simulink model "MODELODETURBINADERIOV5"  (R2017a)
settings: Solver=ode45  StartTime=0.0  StopTime=0.05  FixedStep=50e-3  MaxStep=0.01  RelTol=1e-3
values from neighbouring files (symbols this model uses):
  A = pi()*((D/2)^2)    [MODELOHIDRO.m]    (also in MODELOHIDROV10.m; MODELOHIDROV2.m; MODELOHIDROV3.m; MODELOHIDROV4.m)
  B = 0    [MODELOHIDRO.m]    (also in MODELOHIDROV10.m; MODELOHIDROV2.m; MODELOHIDROV3.m; MODELOHIDROV4.m)
  beta = 0    [MODELOHIDRO.m]    (also in MODELOHIDROV10.m; MODELOHIDROV2.m; MODELOHIDROV3.m; MODELOHIDROV4.m)
  Bi = 0.2287    [MODELOHIDRO.m]    (also in MODELOHIDROV10.m = 0.1; MODELOHIDROV2.m; MODELOHIDROV3.m; MODELOHIDROV4.m = 0.005)
  den = 1000    [MODELOHIDRO.m]    (also in MODELOHIDROV10.m; MODELOHIDROV2.m; MODELOHIDROV3.m; MODELOHIDROV4.m)
  J = 16.1919e-4    (= 0.00161919)    [MODELOHIDROV10.m]    (also in MODELOHIDROV2.m = 100; MODELOHIDROV3.m = 10; MODELOHIDROV4.m; MODELOHIDROV7.m)
  Ji = 1    [MODELOHIDRO.m]    (also in MODELOHIDROV10.m = 1.72; MODELOHIDROV2.m; MODELOHIDROV3.m; MODELOHIDROV4.m = 0.0465)
  Kb = 1.8    [MODELOHIDRO.m]    (also in MODELOHIDROV10.m = 6.2; MODELOHIDROV2.m; MODELOHIDROV3.m; MODELOHIDROV4.m = 0.027)
  Kp = 0.4    [MODELOHIDRO.m]    (also in MODELOHIDROV10.m = 5.6627; MODELOHIDROV2.m; MODELOHIDROV3.m; MODELOHIDROV4.m = 0.027)
  L_d = 38e-3    (= 0.038)    [MODELOHIDROV2.m]    (also in MODELOHIDROV3.m; MODELOHIDROV4.m; MODELOHIDROV7.m)
  L_q = 9.03e-3    (= 0.00903)    [MODELOHIDROV2.m]    (also in MODELOHIDROV3.m; MODELOHIDROV4.m; MODELOHIDROV7.m)
  Lambda = 0.48    [MODELOHIDROV2.m]    (also in MODELOHIDROV3.m; MODELOHIDROV4.m; MODELOHIDROV7.m)
  P = 1    [MODELOHIDROV2.m]    (also in MODELOHIDROV3.m; MODELOHIDROV4.m; MODELOHIDROV7.m)
  r = D/2    (= 0.5)    [MODELOHIDRO.m]    (also in MODELOHIDROV10.m; MODELOHIDROV2.m; MODELOHIDROV3.m; MODELOHIDROV4.m)
  Ri = 0.6    [MODELOHIDRO.m]    (also in MODELOHIDROV10.m = 0.973; MODELOHIDROV2.m; MODELOHIDROV3.m; MODELOHIDROV4.m = 1)
  Rs = 1.649    [MODELOHIDROV2.m]    (also in MODELOHIDROV3.m; MODELOHIDROV4.m; MODELOHIDROV7.m)
  T_d = 0    [MODELOHIDRO.m]    (also in MODELOHIDROV10.m; MODELOHIDROV2.m; MODELOHIDROV3.m; MODELOHIDROV4.m)
undefined symbols (not defined in the file or in its folder): sigbuilder_block
libraries: powerlib x19, simulink x2
settings Model: Creator=zni.uao  LastModifiedBy=zni.uao
settings SolverCC: ZeroCrossAlgorithm=Adaptive
settings OptimizationCC: LifeSpan=inf
settings HardwareCC: ProdBitPerPointer=32  ProdBitPerSizeT=32  ProdBitPerPtrDiffT=32  ProdLargestAtomicFloat=None  ProdWordSize=32  ProdHWDeviceType=Custom Processor->Custom

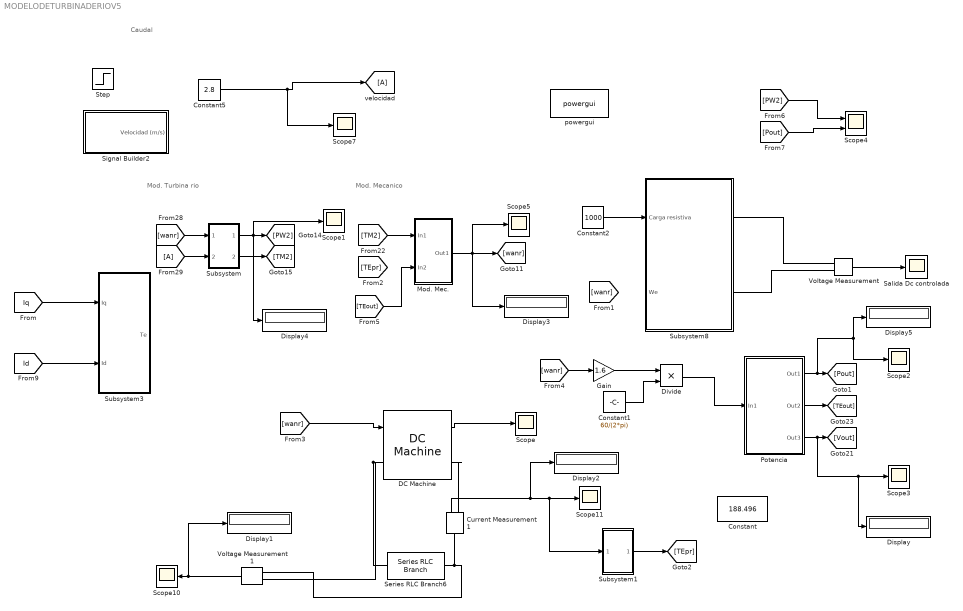
== system MODELODETURBINADERIOV5 ==
  note: Mod. Turbina rio
  note: Mod. Mecanico
  note: Caudal
  Constant : Constant  Value=188.496
  Constant1 : Constant  Value=60/(2*pi)
  Constant2 : Constant  Value=1000
  Constant5 : Constant  Value=2.8
  Current Measurement1 : powerlib/Measurements/Current Measurement  PhasorSimulation=off  OutputType=Complex  PSBequivalent=0
  DC Machine : powerlib/Machines/DC Machine  PresetModel=No  MechanicalLoad=Speed w  FieldType=Permanent magnet  ShowDetailedParameters=on  MeasurementBus=off  RLa=[0.78 0.016]  RLf=[150 112.5]  Laf=1.234  MachineConstant=Torque constant (N.m/A)  Ke=1.8  Kt=1.8  J=0.05  Bm=0.01  Tf=0  w0=1  Ifinit=1  TsPowergui=0  TsBlock=-1
  Display{,1..5} (6 alike) : Display
  Divide : Product  Inputs=**
  Gain : Gain  Gain=1.6
  Mod. Mec. : Subsystem
  Potencia : Subsystem
  Salida Dc controlada : Scope
  Scope{,1..3,5,7,10..11} (8 alike) : Scope
  Scope4 : Scope  NumInputPorts=2
  Series RLC Branch6 : powerlib/Elements/Series RLC Branch  LConnTagsString=__new0  RConnTagsString=__new0  BranchType=R  Resistance=1000  Inductance=1e-3  SetiL0=off  InitialCurrent=0  Capacitance=1e-6  Setx0=off  InitialVoltage=0  Measurements=None
  Signal Builder2 : Subsystem  Tag=STV Subsys  LoadFcn=sigbuilder_block('load');  StartFcn=sigbuilder_block('start');  StopFcn=sigbuilder_block('stop');  ClipboardFcn=sigbuilder_block('clipboard');  mask(Sigbuilder block){tuvar=[0:10]}
      mask help: Simulink:masks:SigbuilderBlock_MD
      mask init:
      | if ~strcmp(get_param(bdroot(gcbh),'SimulationStatus'),'stopped') tuvar = sigbuilder_block('maskInit'); end
      settings: CopyFcn=sigbuilder_block('copy');  DeleteFcn=sigbuilder_block('delete');  ModelCloseFcn=sigbuilder_block('modelClose');  PreSaveFcn=sigbuilder_block('preSave');  PauseFcn=sigbuilder_block('pause');  ContinueFcn=sigbuilder_block('continue');  NameChangeFcn=sigbuilder_block('namechange');  OpenFcn=sigbuilder_block('open',[197.25 66 550.5 359.25 ]);  CloseFcn=sigbuilder_block('close');
      mask Display: plot(0, 0, 100, 100,[2, 2, 32, 32, 2], [68, 8, 8, 68, 68],[32, 2], [38, 38], [32, 19, 2],[53, 60, 44], [32, 17, 17, 2],[16, 16, 31, 31]);txt = getActiveGroup(gcbh);text(2, 100, txt,'verticalAlignment', 'top');
  Step : Step  Time=10  Before=2.5  After=2.888  SampleTime=0
  Subsystem : Subsystem
  Subsystem1 : Subsystem
  Subsystem3 : Subsystem
  Subsystem8 : Subsystem
  Voltage Measurement : powerlib/Measurements/Voltage Measurement  PhasorSimulation=off  OutputType=Complex  PSBequivalent=0
  Voltage Measurement1 : powerlib/Measurements/Voltage Measurement  PhasorSimulation=off  OutputType=Complex  PSBequivalent=0
  powergui : powerlib/powergui  Priority=1  SimulationMode=Continuous  SampleTime=50e-3  frequency=60  Iterations=50  frequencyindice=0  Pbase=100e6  ErrMax=1e-4  UnitsV=kV  UnitsW=MW  buscounter=0  FunctionMessages=off  echomessages=off  EnableUseOfTLC=off  CurrentSourceSwitches=off  DisableSnubberDevices=off  DisableRonSwitches=off  DisableVfSwitches=off  DisplayEquations=off  SolverType=Tustin/Backward Euler (TBE)  Interpol=off  ExternalGateDelay=off  methode=off  Ts=100  x0status=blocks  SPID=off  SwTol=0  HookPort=off  RestoreLinks=warning  ResistiveCurrentMeasurement=off  Frange=[0:2:500]  Ylog=off  Xlog=on  ShowGrid=off  save=off  variable=ZData  structure=0  ZoomFFT=off  StartTime=0.0  cycles=1  DisplayStyle=1  fundamental=60  FreqAxis=off  MaxFrequency=1000  frequencyindicesteady=0 Hz  RmsSteady=1  display=off
  wires:
  [wanr] -> Subsystem/1(In1)
  [A] -> Subsystem/2(In2)
  Subsystem/1(Out1) -> Display4/1, Scope1/1, [PW2]
  Subsystem/2(Out2) -> [TM2]
  Mod. Mec./1(Out1) -> Display3/1, Scope5/1, [wanr]
  [TM2] -> Mod. Mec./1(In1)
  [Iq] -> Subsystem3/1(Iq)
  [Id] -> Subsystem3/2(Id)
  Constant2/1 -> Subsystem8/1(Carga resistiva)
  Voltage Measurement/1 -> Salida Dc controlada/1
  [wanr] -> DC Machine/1
  Voltage Measurement1/1 -> Display1/1, Scope10/1
  DC Machine/1 -> Scope/1
  Current Measurement1/1 -> Display2/1, Subsystem1/1(In1), Scope11/1
  Subsystem1/1(Out1) -> [TEpr]
  Potencia/1(Out1) -> Display5/1, Scope2/1, [Pout]
  Potencia/3(Out3) -> Display/1, Scope3/1, [Vout]
  Potencia/2(Out2) -> [TEout]
  [PW2] -> Scope4/1
  [Pout] -> Scope4/2
  [TEout] -> Mod. Mec./2(In2)
  Constant5/1 -> Scope7/1, [A]
  Gain/1 -> Divide/1
  Constant1/1 -> Divide/2
  Divide/1 -> Potencia/1(In1)
  [wanr] -> Gain/1
  connections:
  Subsystem8/RConn2 -- Voltage Measurement/LConn2
  Subsystem8/RConn1 -- Voltage Measurement/LConn1
  Current Measurement1/LConn1 -- Series RLC Branch6/RConn1 -- Voltage Measurement1/LConn2
  DC Machine/LConn1 -- Series RLC Branch6/LConn1 -- Voltage Measurement1/LConn1
  DC Machine/RConn1 -- Current Measurement1/RConn1

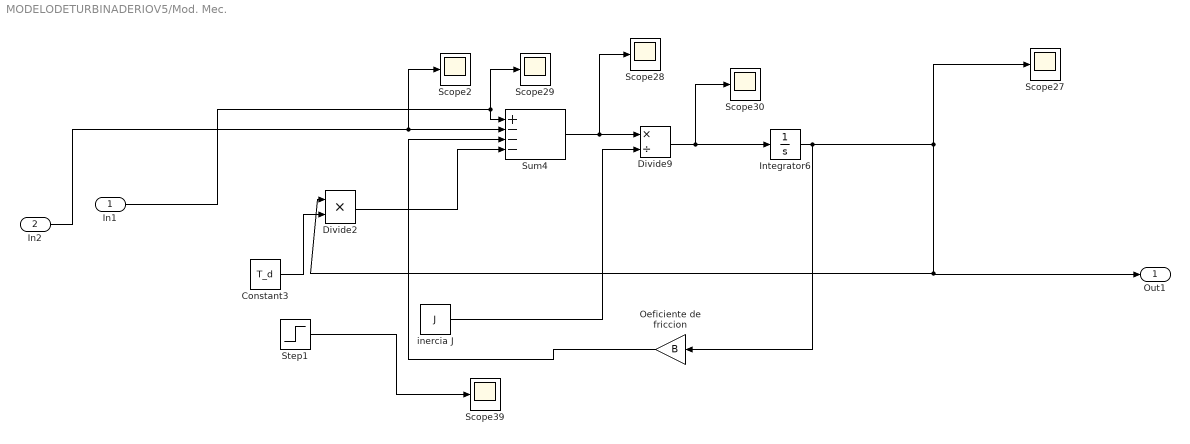
== system MODELODETURBINADERIOV5/Mod. Mec. ==
  In1 : Inport
  In2 : Inport  Port=2
  Constant3 : Constant  Value=T_d
  Divide2 : Product  Inputs=**
  Divide9 : Product  Inputs=*/
  Integrator6 : Integrator  InitialCondition=10
  Oeficiente de friccion : Gain  Gain=B
  Scope{2,27..30,39} (6 alike) : Scope
  Step1 : Step  Time=3  Before=4  After=0  SampleTime=0
  Sum4 : Sum  Inputs=|+---
  inercia J : Constant  Value=J
  Out1 : Outport
  wires:
  inercia J/1 -> Divide9/2
  Constant3/1 -> Divide2/2
  Divide2/1 -> Sum4/4
  Oeficiente de friccion/1 -> Sum4/3
  Step1/1 -> Scope39/1
  Sum4/1 -> Scope28/1, Divide9/1
  In1/1 -> Scope29/1, Sum4/1
  In2/1 -> Scope2/1, Sum4/2
  Divide9/1 -> Scope30/1, Integrator6/1
  Integrator6/1 -> Out1/1, Divide2/1, Scope27/1, Oeficiente de friccion/1

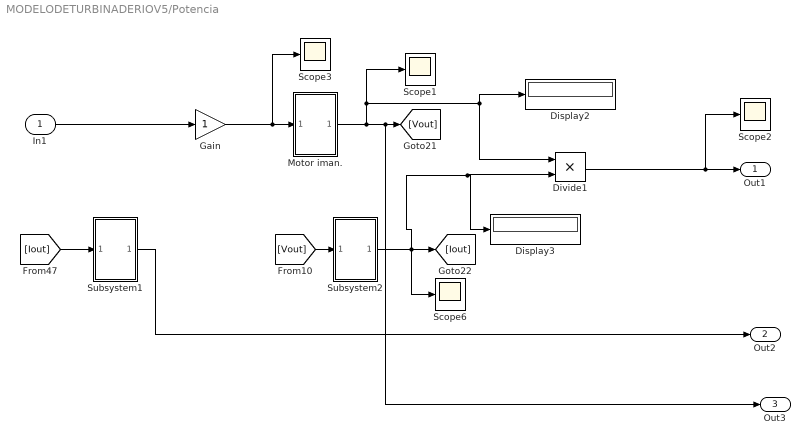
== system MODELODETURBINADERIOV5/Potencia ==
  In1 : Inport
  Display2 : Display
  Display3 : Display
  Divide1 : Product  Inputs=**
  Gain : Gain
  Motor iman. : Subsystem
  Scope{1..3,6} (4 alike) : Scope
  Subsystem1 : Subsystem
  Subsystem2 : Subsystem
  Out1 : Outport
  Out2 : Outport  Port=2
  Out3 : Outport  Port=3
  wires:
  Motor iman./1(Out1) -> Out3/1, [Vout], Scope1/1, Divide1/1, Display2/1
  Subsystem1/1(Out1) -> Out2/1
  [Iout] -> Subsystem1/1(In1)
  Subsystem2/1(Out1) -> Divide1/2, Display3/1, Scope6/1, [Iout]
  Divide1/1 -> Scope2/1, Out1/1
  Gain/1 -> Scope3/1, Motor iman./1(In1)
  In1/1 -> Gain/1
  [Vout] -> Subsystem2/1(In1)

== system MODELODETURBINADERIOV5/Signal Builder2 ==
  Demux : Demux  Tag=STV Demux  Outputs=1
  FromWs : FromWorkspace  Tag=STV FromWs  VariableName=tuvar  SampleTime=0
      SigBuilderData=|
      | common.afterFinalStr = 'Extrapolate'
      | common.sampleTime = 0
      | dataSet.timeRange = [0 0.1]
      | dataSet.name = 'Group 1'
      | sbobj.Groups.Name = 'Group 1'
      | sbobj.Groups.Signals.Name = 'Velocidad (m/s)'
      | sbobj.Groups.Signals.XData = [0 0.01 0.01 0.02 0.02 0.0298 0.0298 0.0398 0.0498 0.06 0.1]
      | sbobj.Groups.Signals.YData = [2 2 2.5 2.5 2.595 2.595 2.8 2.8 2.8 2.8 2.8]
      | sbobj.Groups.TimeRange = [0 0.1]
  Velocidad (m/s) : Outport  Tag=STV Outport
  wires:
  FromWs/1 -> Demux/1
  Demux/1 -> Velocidad (m/s)/1

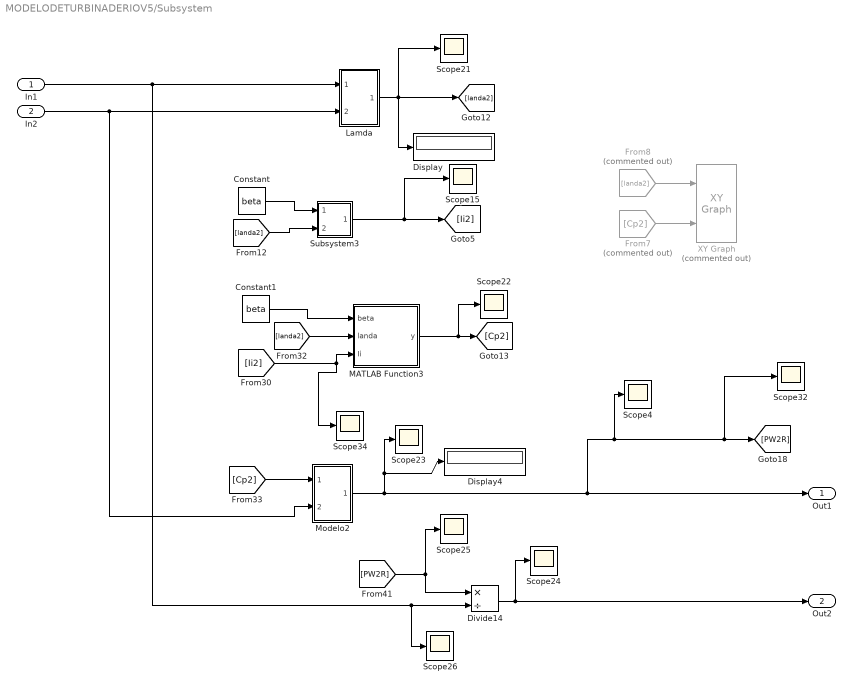
== system MODELODETURBINADERIOV5/Subsystem ==
  In1 : Inport
  In2 : Inport  Port=2
  Constant : Constant  Value=beta
  Constant1 : Constant  Value=beta
  Display : Display
  Display4 : Display
  Divide14 : Product  Inputs=*/
  From7 : From  Commented=on  GotoTag=Cp2
  From8 : From  Commented=on  GotoTag=landa2
  Lamda : Subsystem
  MATLAB Function3 : MATLAB Function  TreatAsAtomicUnit=on
  Modelo2 : Subsystem
  Scope{4,15,21..26,32,34} (10 alike) : Scope
  Subsystem3 : Subsystem
  XY Graph : simulink/Sinks/XY Graph  Commented=on  xmin=1  xmax=20  ymin=0  ymax=0.56  st=0.1
  Out1 : Outport
  Out2 : Outport  Port=2
  wires:
  Constant1/1 -> MATLAB Function3/1(beta)
  Divide14/1 -> Out2/1, Scope24/1
  [Ii2] -> Scope34/1, MATLAB Function3/3(Ii)
  [Cp2] -> Modelo2/1(In1)
  [PW2R] -> Scope25/1, Divide14/1
  In1/1 -> Scope26/1, Divide14/2, Lamda/1(In1)
  [landa2] -> MATLAB Function3/2(landa)
  In2/1 -> Modelo2/2(In2), Lamda/2(In2)
  Lamda/1(Out1) -> Display/1, [landa2], Scope21/1
  MATLAB Function3/1(y) -> Scope22/1, [Cp2]
  From8/1 -> XY Graph/1
  Constant/1 -> Subsystem3/1(In1)
  [landa2] -> Subsystem3/2(In2)
  Modelo2/1(Out1) -> Scope32/1, [PW2R], Scope4/1, Out1/1, Display4/1, Scope23/1
  Subsystem3/1(Out1) -> Scope15/1, [Ii2]
  From7/1 -> XY Graph/2

== system MODELODETURBINADERIOV5/Subsystem1 ==
  In1 : Inport
  Constant2 : Constant  Value=Kp
  Divide2 : Product  Inputs=**
  Out1 : Outport
  wires:
  In1/1 -> Divide2/1
  Constant2/1 -> Divide2/2
  Divide2/1 -> Out1/1

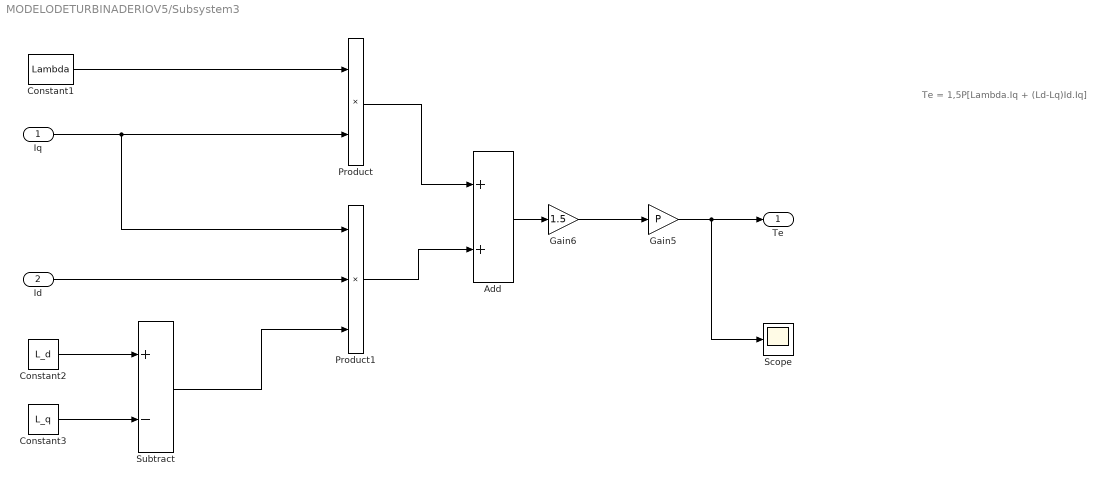
== system MODELODETURBINADERIOV5/Subsystem3 ==
  note: Te = 1,5P[Lambda.Iq + (Ld-Lq)Id.Iq]
  Iq : Inport
  Id : Inport  Port=2
  Add : Sum
  Constant1 : Constant  Value=Lambda
  Constant2 : Constant  Value=L_d
  Constant3 : Constant  Value=L_q
  Gain5 : Gain  Gain=P
  Gain6 : Gain  Gain=1.5
  Product : Product
  Product1 : Product  Inputs=3
  Scope : Scope
  Subtract : Sum  Inputs=+-
  Te : Outport
  wires:
  Product1/1 -> Add/2
  Iq/1 -> Product1/1, Product/2
  Constant1/1 -> Product/1
  Gain5/1 -> Scope/1, Te/1
  Subtract/1 -> Product1/3
  Id/1 -> Product1/2
  Gain6/1 -> Gain5/1
  Add/1 -> Gain6/1
  Product/1 -> Add/1
  Constant2/1 -> Subtract/1
  Constant3/1 -> Subtract/2

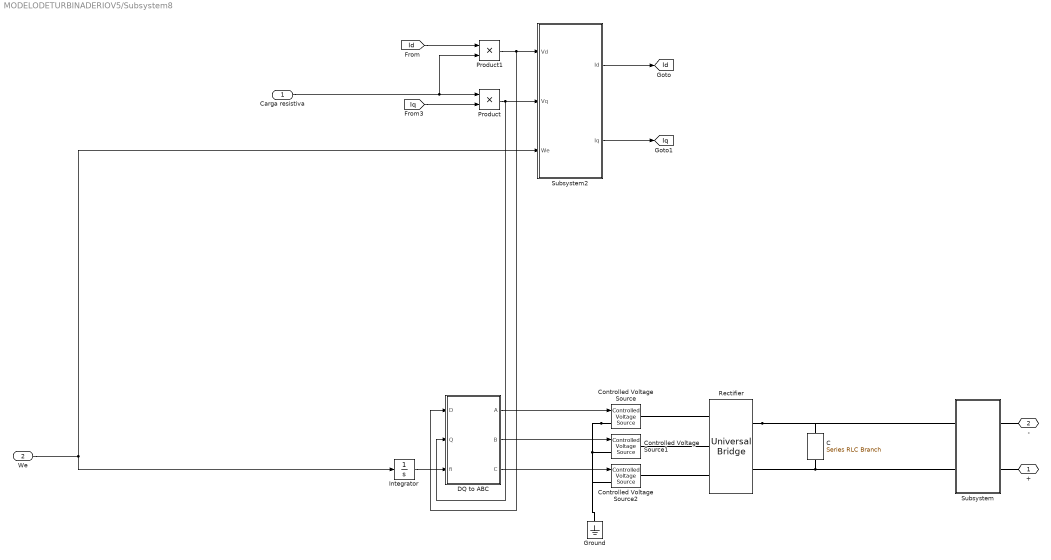
== system MODELODETURBINADERIOV5/Subsystem8 ==
  Carga resistiva : Inport
  We : Inport  Port=2
  C : powerlib/Elements/Series RLC Branch  LConnTagsString=__new0  RConnTagsString=__new0  BranchType=C  Resistance=1e3  Inductance=1e-3  SetiL0=off  InitialCurrent=0  Capacitance=4700e-6  Setx0=off  InitialVoltage=0  Measurements=None
  Controlled Voltage Source : powerlib/Electrical Sources/Controlled Voltage Source  Initialize=off  Source_Type=AC  Amplitude=0  Phase=0  Frequency=0  Measurements=None
  Controlled Voltage Source1 : powerlib/Electrical Sources/Controlled Voltage Source  Initialize=off  Source_Type=AC  Amplitude=0  Phase=0  Frequency=0  Measurements=None
  Controlled Voltage Source2 : powerlib/Electrical Sources/Controlled Voltage Source  Initialize=off  Source_Type=AC  Amplitude=0  Phase=0  Frequency=0  Measurements=None
  DQ to ABC : Subsystem
  Ground : powerlib/Elements/Ground  LConnTagsString=a
  Integrator : Integrator
  Product : Product
  Product1 : Product
  Rectifier : powerlib/Power Electronics/Universal Bridge  Arms=3  SnubberResistance=100  SnubberCapacitance=0.1e-6  Device=Diodes  Ron=1e-3  Lon=0  ForwardVoltages="[  0.8  0.8  ]"  ForwardVoltage=.8  GTOparameters=[ 10e-6 , 20e-6 ]  IGBTparameters=[ 1e-6 , 2e-6 ]  Measurements=Device currents  Measurements_2=None  converterType=Rectifier
  Subsystem : Subsystem
  Subsystem2 : Subsystem
  + : PMIOPort  Port=1  Side=Right
  - : PMIOPort  Port=2  Side=Right
  tag scope: Id=global, Iq=global
  wires:
  [Iq] -> Product/2
  [Id] -> Product1/1
  We/1 -> Subsystem2/3(We), Integrator/1
  Carga resistiva/1 -> Product/1, Product1/2
  Subsystem2/1(Id) -> [Id]
  DQ to ABC/1(A) -> Controlled Voltage Source/1
  DQ to ABC/3(C) -> Controlled Voltage Source2/1
  DQ to ABC/2("B ") -> Controlled Voltage Source1/1
  Subsystem2/2(Iq) -> [Iq]
  Product1/1 -> Subsystem2/1(Vd), DQ to ABC/1(D)
  Product/1 -> Subsystem2/2(Vq), DQ to ABC/2(Q)
  Integrator/1 -> DQ to ABC/3(fi)
  connections:
  Subsystem/RConn1 -- -/RConn1
  Subsystem/RConn2 -- +/RConn1
  Controlled Voltage Source/LConn1 -- Ground/LConn1 -- Controlled Voltage Source2/LConn1 -- Controlled Voltage Source1/LConn1
  Subsystem/LConn2 -- Rectifier/RConn2 -- C/RConn1
  Rectifier/LConn1 -- Controlled Voltage Source/RConn1
  Rectifier/LConn3 -- Controlled Voltage Source2/RConn1
  Rectifier/LConn2 -- Controlled Voltage Source1/RConn1
  Rectifier/RConn1 -- Subsystem/LConn1 -- C/LConn1

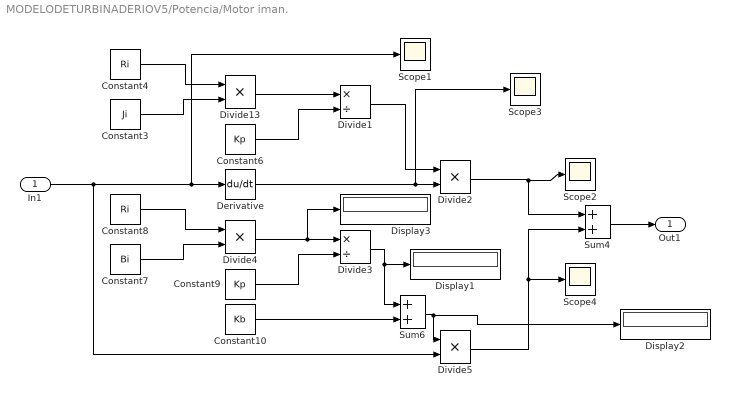
== system MODELODETURBINADERIOV5/Potencia/Motor iman. ==
  In1 : Inport
  Constant10 : Constant  Value=Kb
  Constant3 : Constant  Value=Ji
  Constant4 : Constant  Value=Ri
  Constant6 : Constant  Value=Kp
  Constant7 : Constant  Value=Bi
  Constant8 : Constant  Value=Ri
  Constant9 : Constant  Value=Kp
  Derivative : Derivative
  Display1 : Display
  Display2 : Display
  Display3 : Display
  Divide1 : Product  Inputs=*/  SaturateOnIntegerOverflow=on  RndMeth=Zero
  Divide{2,4..5,13} (4 alike) : Product  Inputs=**  SaturateOnIntegerOverflow=on  RndMeth=Zero
  Divide3 : Product  Inputs=*/  SaturateOnIntegerOverflow=on  RndMeth=Zero
  Scope{1..4} (4 alike) : Scope
  Sum4 : Sum
  Sum6 : Sum
  Out1 : Outport
  wires:
  Constant10/1 -> Sum6/2
  Divide2/1 -> Scope2/1, Sum4/1
  In1/1 -> Divide5/2, Scope1/1, Derivative/1
  Divide3/1 -> Display1/1, Sum6/1
  Divide13/1 -> Divide1/1
  Constant6/1 -> Divide1/2
  Constant4/1 -> Divide13/1
  Sum6/1 -> Display2/1, Divide5/1
  Divide1/1 -> Divide2/1
  Constant3/1 -> Divide13/2
  Constant9/1 -> Divide3/2
  Divide4/1 -> Display3/1, Divide3/1
  Constant7/1 -> Divide4/2
  Constant8/1 -> Divide4/1
  Derivative/1 -> Scope3/1, Divide2/2
  Sum4/1 -> Out1/1
  Divide5/1 -> Scope4/1, Sum4/2

== system MODELODETURBINADERIOV5/Potencia/Subsystem1 ==
  In1 : Inport
  Constant2 : Constant  Value=Kp
  Divide2 : Product  Inputs=**
  Out1 : Outport
  wires:
  In1/1 -> Divide2/1
  Constant2/1 -> Divide2/2
  Divide2/1 -> Out1/1

== system MODELODETURBINADERIOV5/Potencia/Subsystem2 ==
  In1 : Inport
  Constant : Constant  Value=250
  Divide1 : Product  Inputs=*/
  Out1 : Outport
  wires:
  Divide1/1 -> Out1/1
  Constant/1 -> Divide1/2
  In1/1 -> Divide1/1

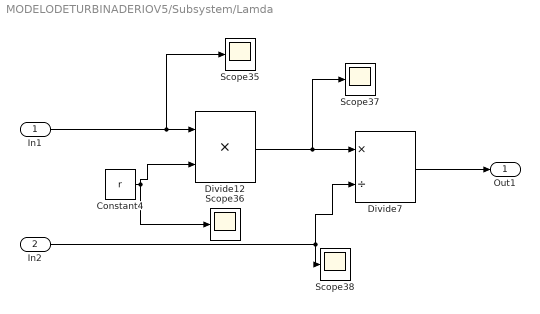
== system MODELODETURBINADERIOV5/Subsystem/Lamda ==
  In1 : Inport
  In2 : Inport  Port=2
  Constant4 : Constant  Value=r
  Divide12 : Product  Inputs=**
  Divide7 : Product  Inputs=*/
  Scope{35..38} (4 alike) : Scope
  Out1 : Outport
  wires:
  Divide7/1 -> Out1/1
  Constant4/1 -> Divide12/2, Scope36/1
  In2/1 -> Divide7/2, Scope38/1
  Divide12/1 -> Scope37/1, Divide7/1
  In1/1 -> Scope35/1, Divide12/1

== system MODELODETURBINADERIOV5/Subsystem/Modelo2 ==
  In1 : Inport
  In2 : Inport  Port=2
  A1 : Constant  Value=A
  Constant4 : Constant  Value=3
  D1 : Constant  Value=den
  Divide13 : Product  Inputs=****  SaturateOnIntegerOverflow=on  RndMeth=Zero
  Gain11 : Gain  Gain=0.5
  Math Function6 : Math  Operator=pow  SaturateOnIntegerOverflow=on
  Out1 : Outport
  wires:
  Constant4/1 -> Math Function6/2
  Divide13/1 -> Gain11/1
  D1/1 -> Divide13/3
  In1/1 -> Divide13/1
  Gain11/1 -> Out1/1
  A1/1 -> Divide13/2
  In2/1 -> Math Function6/1
  Math Function6/1 -> Divide13/4

== system MODELODETURBINADERIOV5/Subsystem/Subsystem3 ==
  In1 : Inport
  In2 : Inport  Port=2
  lamdai : MATLAB Function  TreatAsAtomicUnit=on
  Out1 : Outport
  wires:
  lamdai/1(Ii) -> Out1/1
  In2/1 -> lamdai/2(landa)
  In1/1 -> lamdai/1(beta)

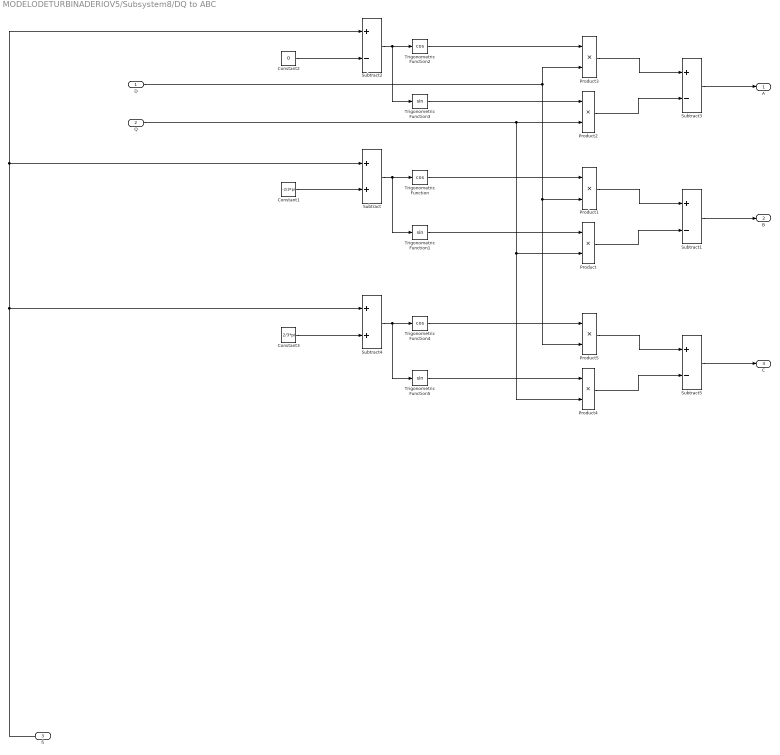
== system MODELODETURBINADERIOV5/Subsystem8/DQ to ABC ==
  D : Inport
  Q : Inport  Port=2
  fi : Inport  Port=3
  Constant1 : Constant  Value=-2/3*pi
  Constant2 : Constant  Value=0
  Constant3 : Constant  Value=2/3*pi
  Product{,1..5} (6 alike) : Product
  Subtract : Sum
  Subtract{1..3,5} (4 alike) : Sum  Inputs=+-
  Subtract4 : Sum
  Trigonometric Function : Trigonometry  Operator=cos
  Trigonometric Function1 : Trigonometry
  Trigonometric Function2 : Trigonometry  Operator=cos
  Trigonometric Function3 : Trigonometry
  Trigonometric Function4 : Trigonometry  Operator=cos
  Trigonometric Function5 : Trigonometry
  A : Outport
  "B " : Outport  Port=2
  C : Outport  Port=3
  wires:
  D/1 -> Product1/2, Product5/2, Product3/2
  Trigonometric Function2/1 -> Product3/1
  Product3/1 -> Subtract3/1
  Subtract3/1 -> A/1
  Subtract2/1 -> Trigonometric Function3/1, Trigonometric Function2/1
  Trigonometric Function3/1 -> Product2/1
  Product2/1 -> Subtract3/2
  Constant2/1 -> Subtract2/2
  Q/1 -> Product2/2, Product4/2, Product/2
  Product/1 -> Subtract1/2
  Subtract1/1 -> "B "/1
  Trigonometric Function/1 -> Product1/1
  Trigonometric Function1/1 -> Product/1
  Product4/1 -> Subtract5/2
  Product5/1 -> Subtract5/1
  Trigonometric Function4/1 -> Product5/1
  Trigonometric Function5/1 -> Product4/1
  Constant3/1 -> Subtract4/2
  Subtract4/1 -> Trigonometric Function5/1, Trigonometric Function4/1
  Subtract5/1 -> C/1
  Product1/1 -> Subtract1/1
  Constant1/1 -> Subtract/2
  Subtract/1 -> Trigonometric Function/1, Trigonometric Function1/1
  fi/1 -> Subtract/1, Subtract2/1, Subtract4/1

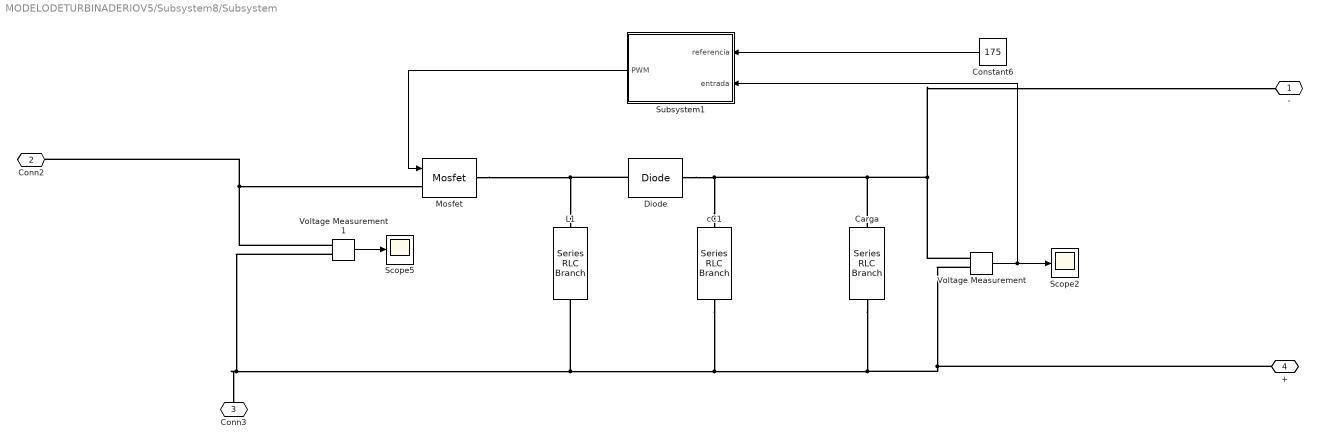
== system MODELODETURBINADERIOV5/Subsystem8/Subsystem ==
  Carga : powerlib/Elements/Series RLC Branch  LConnTagsString=__new0  RConnTagsString=__new0  BranchType=R  Resistance=500  Inductance=1e-3  SetiL0=off  InitialCurrent=0  Capacitance=1e-6  Setx0=off  InitialVoltage=0  Measurements=None
  Constant6 : Constant  Value=175
  Diode : powerlib/Power Electronics/Diode  Ron=0.001  Lon=0  Vf=0.8  IC=0  UseSnubber=off  Rs=500  Cs=250e-9  Measurements=off
  L1 : powerlib/Elements/Series RLC Branch  LConnTagsString=__new0  RConnTagsString=__new0  BranchType=L  Resistance=1  Inductance=428.99e-6  SetiL0=off  InitialCurrent=0  Capacitance=1e-6  Setx0=off  InitialVoltage=0  Measurements=None
  Mosfet : powerlib/Power Electronics/Mosfet  Ron=0.1  Lon=0  Rd=0.01  Vfd=0  IC=0  Rs=1e5  Cs=inf  Measurements=off
  Scope2 : Scope
  Scope5 : Scope
  Subsystem1 : Subsystem
  Voltage Measurement : powerlib/Measurements/Voltage Measurement  PhasorSimulation=off  OutputType=Complex  PSBequivalent=0
  Voltage Measurement1 : powerlib/Measurements/Voltage Measurement  PhasorSimulation=off  OutputType=Complex  PSBequivalent=0
  cC1 : powerlib/Elements/Series RLC Branch  LConnTagsString=__new0  RConnTagsString=__new0  BranchType=C  Resistance=1  Inductance=1e-3  SetiL0=off  InitialCurrent=0  Capacitance=6200e-6  Setx0=off  InitialVoltage=0  Measurements=None
  - : PMIOPort  Port=1  Side=Right
  Conn2 : PMIOPort  Port=2  Side=Left
  Conn3 : PMIOPort  Port=3  Side=Left
  + : PMIOPort  Port=4  Side=Right
  wires:
  Voltage Measurement1/1 -> Scope5/1
  Constant6/1 -> Subsystem1/1(referencia)
  Subsystem1/1("PWM ") -> Mosfet/1
  Voltage Measurement/1 -> Scope2/1, Subsystem1/2(entrada)
  connections:
  cC1/LConn1 -- Diode/LConn1 -- Carga/LConn1 -- -/RConn1 -- Voltage Measurement/LConn1
  Voltage Measurement1/LConn1 -- Conn2/RConn1 -- Mosfet/LConn1
  L1/RConn1 -- cC1/RConn1 -- Carga/RConn1 -- Voltage Measurement/LConn2 -- +/RConn1 -- Conn3/RConn1 -- Voltage Measurement1/LConn2
  Mosfet/RConn1 -- Diode/RConn1 -- L1/LConn1

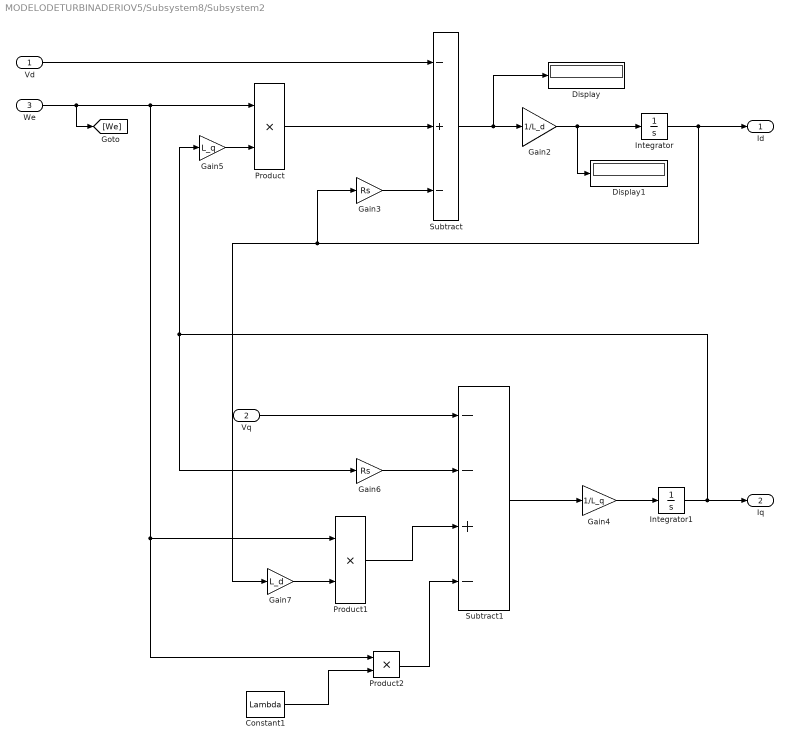
== system MODELODETURBINADERIOV5/Subsystem8/Subsystem2 ==
  Vd : Inport
  Vq : Inport  Port=2
  We : Inport  Port=3
  Constant1 : Constant  Value=Lambda
  Display : Display
  Display1 : Display
  Gain2 : Gain  Gain=1/L_d
  Gain3 : Gain  Gain=Rs
  Gain4 : Gain  Gain=1/L_q
  Gain5 : Gain  Gain=L_q
  Gain6 : Gain  Gain=Rs
  Gain7 : Gain  Gain=L_d
  Integrator : Integrator
  Integrator1 : Integrator
  Product : Product
  Product1 : Product
  Product2 : Product
  Subtract : Sum  Inputs=-+-
  Subtract1 : Sum  Inputs=--+-
  Id : Outport
  Iq : Outport  Port=2
  wires:
  Gain3/1 -> Subtract/3
  Product2/1 -> Subtract1/4
  Constant1/1 -> Product2/2
  Vd/1 -> Subtract/1
  Gain6/1 -> Subtract1/2
  Vq/1 -> Subtract1/1
  Subtract1/1 -> Gain4/1
  Subtract/1 -> Gain2/1, Display/1
  Gain5/1 -> Product/2
  Gain2/1 -> Integrator/1, Display1/1
  Gain4/1 -> Integrator1/1
  Integrator/1 -> Gain3/1, Gain7/1, Id/1
  Product/1 -> Subtract/2
  Gain7/1 -> Product1/2
  Product1/1 -> Subtract1/3
  We/1 -> Product1/1, Product2/1, Product/1, [We]
  Integrator1/1 -> Iq/1, Gain5/1, Gain6/1

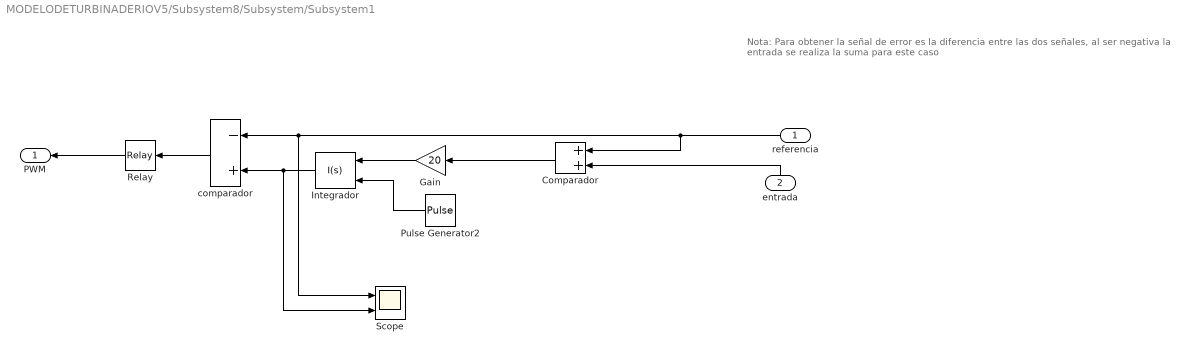
== system MODELODETURBINADERIOV5/Subsystem8/Subsystem/Subsystem1 ==
  note: Nota: Para obtener la señal de error es la
      | diferencia entre las dos señales, al ser negativa
      | la entrada se realiza la suma para este caso
  referencia : Inport
  entrada : Inport  Port=2
  Comparador : Sum
  Gain : Gain  Gain=20
  Integrador : simulink/Continuous/PID Controller  Controller=I  TimeDomain=Continuous-time  SampleTime=-1  IntegratorMethod=Forward Euler  FilterMethod=Forward Euler  Form=Parallel  UseFilter=on  ControllerParametersSource=internal  P=1  I=100e3  D=0  N=100  InitialConditionSource=internal  InitialConditionForIntegrator=0  InitialConditionForFilter=0  ExternalReset=rising  LimitOutput=off  UpperSaturationLimit=inf  LowerSaturationLimit=-inf  LinearizeAsGain=on  AntiWindupMode=none  Kb=1  TrackingMode=off  Kt=1  PParamMin=[]  PParamMax=[]  IParamMin=[]  IParamMax=[]  DParamMin=[]  DParamMax=[]  NParamMin=[]  NParamMax=[]  KbParamMin=[]  KbParamMax=[]  KtParamMin=[]  KtParamMax=[]  POutMin=[]  POutMax=[]  IOutMin=[]  IOutMax=[]  DOutMin=[]  DOutMax=[]  NOutMin=[]  NOutMax=[]  KbOutMin=[]  KbOutMax=[]  KtOutMin=[]  KtOutMax=[]  IntegratorOutMin=[]  IntegratorOutMax=[]  FilterOutMin=[]  FilterOutMax=[]  SumOutMin=[]  SumOutMax=[]  SumI1OutMin=[]  SumI1OutMax=[]  SumI2OutMin=[]  SumI2OutMax=[]  SumI3OutMin=[]  SumI3OutMax=[]  SumDOutMin=[]  SumDOutMax=[]  SaturationOutMin=[]  SaturationOutMax=[]  IntegratorContinuousStateAttributes=''  IntegratorStateMustResolveToSignalObject=off  IntegratorRTWStateStorageClass=Auto  FilterContinuousStateAttributes=''  FilterStateMustResolveToSignalObject=off  FilterRTWStateStorageClass=Auto  DifferentiatorICPrevScaledInput=0  DifferentiatorOutMin=[]  DifferentiatorOutMax=[]  InitialConditionSetting=State (most efficient)
  Pulse Generator2 : DiscretePulseGenerator  PulseType=Time based  Period=40e-6  PulseWidth=50
  Relay : Relay
  Scope : Scope  NumInputPorts=2
  "comparador " : Sum  Inputs=-+
  "PWM " : Outport
  wires:
  Comparador/1 -> Gain/1
  "comparador "/1 -> Relay/1
  entrada/1 -> Comparador/2
  Relay/1 -> "PWM "/1
  Integrador/1 -> "comparador "/2, Scope/2
  Gain/1 -> Integrador/1
  referencia/1 -> Comparador/1, "comparador "/1, Scope/1
  Pulse Generator2/1 -> Integrador/2

== matlab function MODELODETURBINADERIOV5/Subsystem/MATLAB Function3 ==
  data: beta input; y output; landa input; Ii input
function y = fcn(beta, landa,Ii)
w=0.5176; 
w1=116/Ii;
 w2=0.4*beta;
 w3=exp(-21/Ii);
 
 cp=w*(w1-w2-5)*w3+0.0068*landa;
 
 
 
 
 
y=cp;

== matlab function MODELODETURBINADERIOV5/Subsystem/Subsystem3/lamdai ==
  data: beta input; Ii output; landa input
function Ii = fcn(beta,landa)


Iii=(1/((landa+(0.08*beta))))-((0.035)/((beta^3)+1));
Ii=1/Iii;
